simulink model "bms_final_sims_06"  (R2017b)
settings: Solver=VariableStepAuto  StartTime=0.0  StopTime=600  MaxStep=1e-4  RelTol=1e-3
undefined symbols (not defined in the file): DiscIntNeverNeededParam, Ion, Lithium, Ts_Control
libraries: powerlib x61, simulink x20, powerlib_meascontrol x3, simulink_extras x1, electricdrivelib x1
(part 2 of 2)

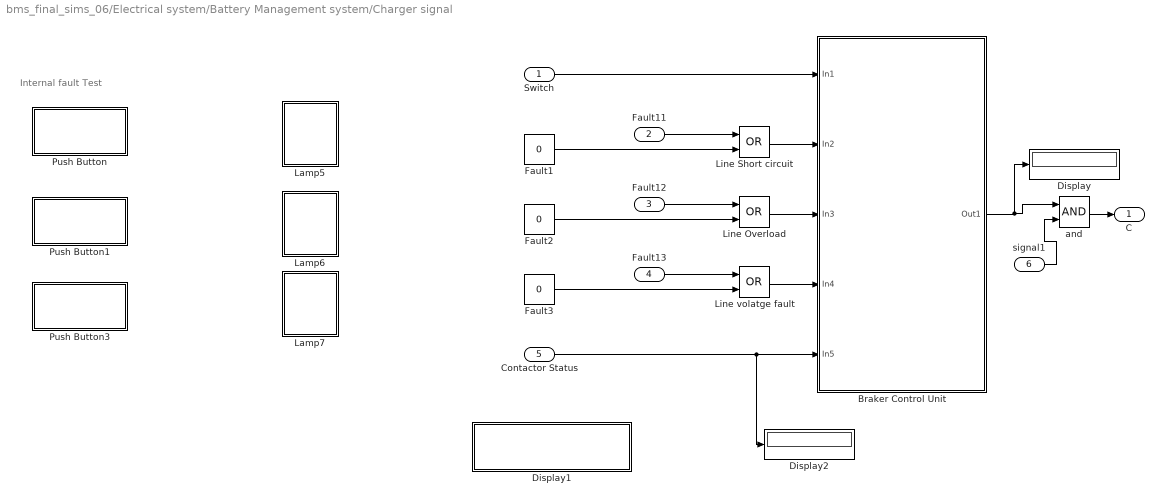
== system bms_final_sims_06/Electrical system/Battery Management system/Charger signal ==
  note: Internal fault Test
  Switch : Inport
  Fault11 : Inport  Port=2
  Fault12 : Inport  Port=3
  Fault13 : Inport  Port=4
  Contactor Status : Inport  Port=5
  signal1 : Inport  Port=6
  Braker Control Unit : Subsystem
  Display : Display
  Display1 : Subsystem  Description=Replaced Block  mask(Replaced Block){}
      mask help: This block has been replaced with an empty subsystem because it used functionality that is unavailable in Simulink R2016b.
      mask Display: fprintf('Replaced: %s\n','Dashboard Widget')
  Display2 : Display
  Fault1 : Constant  Value=0
  Fault2 : Constant  Value=0
  "Fault3 " : Constant  Value=0
  Lamp5 : Subsystem  DialogController=hmiCreateDDGDialog  IsWebBlock=on  mask(MWDashboardBlock){webBlockId=fb817cf7-7d11-4fa1-9a30-af3dbf48badf, webBlockType=lamp, ShowInLibBrowser=on, ShowInitialText=on, HMISrcModelName=bms_final_sims_06}
      mask prompts: webBlockType "WebBlock Type"; HMISrcModelName "Source Model"
      mask help: SimulinkHMI:dialogs:LampDialogDesc
      mask Help: helpview([docroot '/mapfiles/simulink.map'], 'hmi_lamp')
      mask Display:
      | if strcmp(get_param(bdroot(gcb),'BlockDiagramType'), 'library')
      |     image([(matlabroot) '/toolbox/simulink/hmi/icons/Lamp.png']);
      | end
  Lamp6 : Subsystem  DialogController=hmiCreateDDGDialog  IsWebBlock=on  mask(MWDashboardBlock){webBlockId=563e6533-b052-43b9-9c37-f49819595058, webBlockType=lamp, ShowInLibBrowser=on, ShowInitialText=on, HMISrcModelName=bms_final_sims_06}
      mask prompts: webBlockType "WebBlock Type"; HMISrcModelName "Source Model"
      mask help: SimulinkHMI:dialogs:LampDialogDesc
      mask Help: helpview([docroot '/mapfiles/simulink.map'], 'hmi_lamp')
      mask Display:
      | if strcmp(get_param(bdroot(gcb),'BlockDiagramType'), 'library')
      |     image([(matlabroot) '/toolbox/simulink/hmi/icons/Lamp.png']);
      | end
  Lamp7 : Subsystem  DialogController=hmiCreateDDGDialog  IsWebBlock=on  mask(MWDashboardBlock){webBlockId=1f8cf103-18fe-43eb-9390-d12ecce520ad, webBlockType=lamp, ShowInLibBrowser=on, ShowInitialText=on, HMISrcModelName=bms_final_sims_06}
      mask prompts: webBlockType "WebBlock Type"; HMISrcModelName "Source Model"
      mask help: SimulinkHMI:dialogs:LampDialogDesc
      mask Help: helpview([docroot '/mapfiles/simulink.map'], 'hmi_lamp')
      mask Display:
      | if strcmp(get_param(bdroot(gcb),'BlockDiagramType'), 'library')
      |     image([(matlabroot) '/toolbox/simulink/hmi/icons/Lamp.png']);
      | end
  Line Overload : Logic  Operator=OR  AllPortsSameDT=off  OutDataTypeStr=boolean
  Line Short circuit : Logic  Operator=OR  AllPortsSameDT=off  OutDataTypeStr=boolean
  Line volatge fault : Logic  Operator=OR  AllPortsSameDT=off  OutDataTypeStr=boolean
  Push Button : Subsystem  DialogController=hmiCreateDDGDialog  IsWebBlock=on  mask(MWDashboardBlock){webBlockId=7db8609d-5c17-4c61-9b24-8432e4b46d1c, webBlockType=pushbutton, ShowInLibBrwoser=on, ShowInitialText=on, HMISrcModelName=bms_final_sims_06}
      mask prompts: webBlockId "WebBlock Id"; webBlockType "WebBlock Type"; HMISrcModelName "Source Model"
      mask help: SimulinkHMI:dialogs:PushButtonDialogDesc
      mask Help: helpview([docroot '/mapfiles/simulink.map'], 'hmi_push_button')
      mask Display:
      | model = bdroot(gcb);
      | if strcmp(get_param(model,'BlockDiagramType'), 'library')
      |     image([(matlabroot) '/toolbox/simulink/hmi/icons/PushButton.png']);
      | end
  Push Button1 : Subsystem  DialogController=hmiCreateDDGDialog  IsWebBlock=on  mask(MWDashboardBlock){webBlockId=5bbde567-ebf7-4148-9d5e-f5393281e34a, webBlockType=pushbutton, ShowInLibBrwoser=on, ShowInitialText=on, HMISrcModelName=bms_final_sims_06}
      mask prompts: webBlockId "WebBlock Id"; webBlockType "WebBlock Type"; HMISrcModelName "Source Model"
      mask help: SimulinkHMI:dialogs:PushButtonDialogDesc
      mask Help: helpview([docroot '/mapfiles/simulink.map'], 'hmi_push_button')
      mask Display:
      | model = bdroot(gcb);
      | if strcmp(get_param(model,'BlockDiagramType'), 'library')
      |     image([(matlabroot) '/toolbox/simulink/hmi/icons/PushButton.png']);
      | end
  Push Button3 : Subsystem  DialogController=hmiCreateDDGDialog  IsWebBlock=on  mask(MWDashboardBlock){webBlockId=33bc8603-89d5-4b36-aa7c-12e4dfbd94cd, webBlockType=pushbutton, ShowInLibBrwoser=on, ShowInitialText=on, HMISrcModelName=bms_final_sims_06}
      mask prompts: webBlockId "WebBlock Id"; webBlockType "WebBlock Type"; HMISrcModelName "Source Model"
      mask help: SimulinkHMI:dialogs:PushButtonDialogDesc
      mask Help: helpview([docroot '/mapfiles/simulink.map'], 'hmi_push_button')
      mask Display:
      | model = bdroot(gcb);
      | if strcmp(get_param(model,'BlockDiagramType'), 'library')
      |     image([(matlabroot) '/toolbox/simulink/hmi/icons/PushButton.png']);
      | end
  and : Logic  AllPortsSameDT=off  OutDataTypeStr=boolean
  C : Outport
  wires:
  Switch/1 -> Braker Control Unit/1(In1)
  Braker Control Unit/1(Out1) -> and/1, Display/1
  Contactor Status/1 -> Display2/1, Braker Control Unit/5(In5)
  Line Short circuit/1 -> Braker Control Unit/2(In2)
  Line Overload/1 -> Braker Control Unit/3(In3)
  Line volatge fault/1 -> Braker Control Unit/4(In4)
  "Fault3 "/1 -> Line volatge fault/2
  Fault2/1 -> Line Overload/2
  Fault1/1 -> Line Short circuit/2
  Fault11/1 -> Line Short circuit/1
  Fault12/1 -> Line Overload/1
  Fault13/1 -> Line volatge fault/1
  and/1 -> C/1
  signal1/1 -> and/2

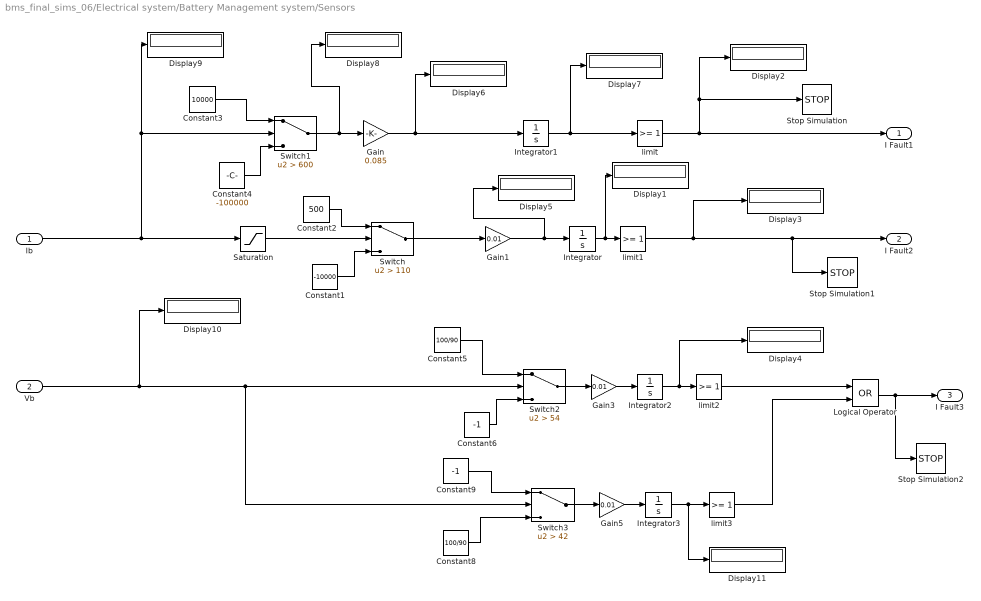
== system bms_final_sims_06/Electrical system/Battery Management system/Sensors ==
  Ib : Inport
  Vb : Inport  Port=2
  Constant1 : Constant  Value=-10000
  Constant2 : Constant  Value=500
  Constant3 : Constant  Value=10000
  Constant4 : Constant  Value=-100000
  Constant5 : Constant  Value=100/90
  Constant6 : Constant  Value=-1
  Constant8 : Constant  Value=100/90
  Constant9 : Constant  Value=-1
  Display{1..11} (11 alike) : Display
  Gain : Gain  Gain=0.085
  Gain1 : Gain  Gain=0.01
  Gain3 : Gain  Gain=0.01
  Gain5 : Gain  Gain=0.01
  Integrator{,1..3} (4 alike) : Integrator  LimitOutput=on  UpperSaturationLimit=1  LowerSaturationLimit=0
  Logical Operator : Logic  Operator=OR  AllPortsSameDT=off  OutDataTypeStr=boolean
  Saturation : Saturate  UpperLimit=600  LowerLimit=-1
  Stop Simulation : Stop
  Stop Simulation1 : Stop
  Stop Simulation2 : Stop
  Switch : Switch  Criteria=u2 > Threshold  Threshold=110
  Switch1 : Switch  Criteria=u2 > Threshold  Threshold=600
  Switch2 : Switch  Criteria=u2 > Threshold  Threshold=54
  Switch3 : Switch  Criteria=u2 > Threshold  Threshold=42
  limit{,1..3} (4 alike) : simulink/Logic and Bit Operations/Compare To Constant  relop=>=  const=1  OutDataTypeStr=boolean
  I Fault1 : Outport
  I Fault2 : Outport  Port=2
  I Fault3 : Outport  Port=3
  wires:
  limit/1 -> I Fault1/1, Stop Simulation/1, Display2/1
  limit1/1 -> Display3/1, I Fault2/1, Stop Simulation1/1
  Integrator/1 -> Display1/1, limit1/1
  Switch/1 -> Gain1/1
  Constant1/1 -> Switch/3
  Integrator1/1 -> Display7/1, limit/1
  Constant3/1 -> Switch1/1
  Gain1/1 -> Display5/1, Integrator/1
  Saturation/1 -> Switch/2
  Constant2/1 -> Switch/1
  Switch1/1 -> Display8/1, Gain/1
  Constant4/1 -> Switch1/3
  Ib/1 -> Saturation/1, Display9/1, Switch1/2
  Gain/1 -> Integrator1/1, Display6/1
  limit2/1 -> Logical Operator/1
  Constant8/1 -> Switch3/3
  Gain5/1 -> Integrator3/1
  Switch3/1 -> Gain5/1
  Integrator2/1 -> Display4/1, limit2/1
  Gain3/1 -> Integrator2/1
  Logical Operator/1 -> I Fault3/1, Stop Simulation2/1
  Switch2/1 -> Gain3/1
  Constant5/1 -> Switch2/1
  Constant6/1 -> Switch2/3
  Constant9/1 -> Switch3/1
  Vb/1 -> Display10/1, Switch3/2, Switch2/2
  Integrator3/1 -> Display11/1, limit3/1
  limit3/1 -> Logical Operator/2

== system bms_final_sims_06/Electrical system/Battery Pack/Battery Cell Equivalent ==
  t : Inport
  Battery : electricdrivelib/Extra Sources/Battery  BatType=Lithium-Ion  ShowTempParam=on  ThermalPreset=no  ShowAgeParam=off  NomV=48  NomQ=100  SOC=62.32  Batt_Tr=30  PresetModel=on  MaxQ=100  MinV=36  FullV=55.8714  Dis_rate=43.4783  R=0.0048  Normal_OP=90.4348  expZone="[51.8585      4.91304]"  current=[6.5 13 32.5]  Units=Time  Tci=20  NomT=20  T2=-30  MaxQ2=4.8  FullV2=7.1  Normal_OP2=5.655  expZone2="[6.58           1]"  Rca=0.6  ti=2000  Dp=0  Neq0=0  Tsim=1e6  Ta1=25  Qeol=5.4*0.9  Reol=0.013333*1.2  Char_age=[2.3478, 3]  Dis_age=[2.3478, 10]  N1=1500  N2=10500  N3=1000  N4=1400  Ta2=45  N5=950
  + : PMIOPort  Port=1  Side=Left
  - : PMIOPort  Port=2  Side=Left
  M : Outport
  wires:
  t/1 -> Battery/1
  Battery/1 -> M/1
  connections:
  Battery/LConn1 -- +/RConn1
  Battery/LConn2 -- -/RConn1

== system bms_final_sims_06/Electrical system/Dashboard Test/Total Fault Test ==
  note: External fault Test
  note: Internal fault Test
  Display : DisplayBlock  WebBlockId=825  ModelName=bms_final_sims_06  LabelPosition=Bottom  ShowInitialText=on  ShowFormattedStrings=off  Format=long  Alignment=Center
  Lamp : Subsystem  DialogController=hmiCreateDDGDialog  IsWebBlock=on  mask(MWDashboardBlock){webBlockId=fbdaa764-5bdc-4e5b-b7dd-49ea15c45a46, webBlockType=lamp, ShowInLibBrowser=on, ShowInitialText=on, HMISrcModelName=bms_final_sims_06}
      mask prompts: webBlockType "WebBlock Type"; HMISrcModelName "Source Model"
      mask help: SimulinkHMI:dialogs:LampDialogDesc
      mask Help: helpview([docroot '/mapfiles/simulink.map'], 'hmi_lamp')
      mask Display:
      | if strcmp(get_param(bdroot(gcb),'BlockDiagramType'), 'library')
      |     image([(matlabroot) '/toolbox/simulink/hmi/icons/Lamp.png']);
      | end
  Lamp1 : Subsystem  DialogController=hmiCreateDDGDialog  IsWebBlock=on  mask(MWDashboardBlock){webBlockId=082af06e-be4e-4919-b618-5f4e7f2fdde3, webBlockType=lamp, ShowInLibBrowser=on, ShowInitialText=on, HMISrcModelName=bms_final_sims_06}
      mask prompts: webBlockType "WebBlock Type"; HMISrcModelName "Source Model"
      mask help: SimulinkHMI:dialogs:LampDialogDesc
      mask Help: helpview([docroot '/mapfiles/simulink.map'], 'hmi_lamp')
      mask Display:
      | if strcmp(get_param(bdroot(gcb),'BlockDiagramType'), 'library')
      |     image([(matlabroot) '/toolbox/simulink/hmi/icons/Lamp.png']);
      | end
  Lamp2 : Subsystem  DialogController=hmiCreateDDGDialog  IsWebBlock=on  mask(MWDashboardBlock){webBlockId=516aa056-5fa7-4a7c-a023-c0dda198eca7, webBlockType=lamp, ShowInLibBrowser=on, ShowInitialText=on, HMISrcModelName=bms_final_sims_06}
      mask prompts: webBlockType "WebBlock Type"; HMISrcModelName "Source Model"
      mask help: SimulinkHMI:dialogs:LampDialogDesc
      mask Help: helpview([docroot '/mapfiles/simulink.map'], 'hmi_lamp')
      mask Display:
      | if strcmp(get_param(bdroot(gcb),'BlockDiagramType'), 'library')
      |     image([(matlabroot) '/toolbox/simulink/hmi/icons/Lamp.png']);
      | end
  Lamp3 : Subsystem  DialogController=hmiCreateDDGDialog  IsWebBlock=on  mask(MWDashboardBlock){webBlockId=fb978a94-c851-419f-aa5a-fdbf15f69119, webBlockType=lamp, ShowInLibBrowser=on, ShowInitialText=on, HMISrcModelName=bms_final_sims_06}
      mask prompts: webBlockType "WebBlock Type"; HMISrcModelName "Source Model"
      mask help: SimulinkHMI:dialogs:LampDialogDesc
      mask Help: helpview([docroot '/mapfiles/simulink.map'], 'hmi_lamp')
      mask Display:
      | if strcmp(get_param(bdroot(gcb),'BlockDiagramType'), 'library')
      |     image([(matlabroot) '/toolbox/simulink/hmi/icons/Lamp.png']);
      | end
  Lamp5 : Subsystem  DialogController=hmiCreateDDGDialog  IsWebBlock=on  mask(MWDashboardBlock){webBlockId=9848dc69-0a60-4163-96c5-d44da9eebd8e, webBlockType=lamp, ShowInLibBrowser=on, ShowInitialText=on, HMISrcModelName=bms_final_sims_06}
      mask prompts: webBlockType "WebBlock Type"; HMISrcModelName "Source Model"
      mask help: SimulinkHMI:dialogs:LampDialogDesc
      mask Help: helpview([docroot '/mapfiles/simulink.map'], 'hmi_lamp')
      mask Display:
      | if strcmp(get_param(bdroot(gcb),'BlockDiagramType'), 'library')
      |     image([(matlabroot) '/toolbox/simulink/hmi/icons/Lamp.png']);
      | end
  Lamp6 : Subsystem  DialogController=hmiCreateDDGDialog  IsWebBlock=on  mask(MWDashboardBlock){webBlockId=70f12f9c-07c1-4b6f-9ffa-b598c3129aa2, webBlockType=lamp, ShowInLibBrowser=on, ShowInitialText=on, HMISrcModelName=bms_final_sims_06}
      mask prompts: webBlockType "WebBlock Type"; HMISrcModelName "Source Model"
      mask help: SimulinkHMI:dialogs:LampDialogDesc
      mask Help: helpview([docroot '/mapfiles/simulink.map'], 'hmi_lamp')
      mask Display:
      | if strcmp(get_param(bdroot(gcb),'BlockDiagramType'), 'library')
      |     image([(matlabroot) '/toolbox/simulink/hmi/icons/Lamp.png']);
      | end
  Lamp7 : Subsystem  DialogController=hmiCreateDDGDialog  IsWebBlock=on  mask(MWDashboardBlock){webBlockId=49f89a92-cf53-4015-be2c-2362d2c7dbc5, webBlockType=lamp, ShowInLibBrowser=on, ShowInitialText=on, HMISrcModelName=bms_final_sims_06}
      mask prompts: webBlockType "WebBlock Type"; HMISrcModelName "Source Model"
      mask help: SimulinkHMI:dialogs:LampDialogDesc
      mask Help: helpview([docroot '/mapfiles/simulink.map'], 'hmi_lamp')
      mask Display:
      | if strcmp(get_param(bdroot(gcb),'BlockDiagramType'), 'library')
      |     image([(matlabroot) '/toolbox/simulink/hmi/icons/Lamp.png']);
      | end
  Push Button : Subsystem  DialogController=hmiCreateDDGDialog  IsWebBlock=on  mask(MWDashboardBlock){webBlockId=516cc25e-937b-498b-86c1-8ec3105bf36c, webBlockType=pushbutton, ShowInLibBrwoser=on, ShowInitialText=on, HMISrcModelName=bms_final_sims_06}
      mask prompts: webBlockId "WebBlock Id"; webBlockType "WebBlock Type"; HMISrcModelName "Source Model"
      mask help: SimulinkHMI:dialogs:PushButtonDialogDesc
      mask Help: helpview([docroot '/mapfiles/simulink.map'], 'hmi_push_button')
      mask Display:
      | model = bdroot(gcb);
      | if strcmp(get_param(model,'BlockDiagramType'), 'library')
      |     image([(matlabroot) '/toolbox/simulink/hmi/icons/PushButton.png']);
      | end
  Push Button1 : Subsystem  DialogController=hmiCreateDDGDialog  IsWebBlock=on  mask(MWDashboardBlock){webBlockId=e4ba1e2c-2ce9-46bd-ab8a-cd5544a9ea11, webBlockType=pushbutton, ShowInLibBrwoser=on, ShowInitialText=on, HMISrcModelName=bms_final_sims_06}
      mask prompts: webBlockId "WebBlock Id"; webBlockType "WebBlock Type"; HMISrcModelName "Source Model"
      mask help: SimulinkHMI:dialogs:PushButtonDialogDesc
      mask Help: helpview([docroot '/mapfiles/simulink.map'], 'hmi_push_button')
      mask Display:
      | model = bdroot(gcb);
      | if strcmp(get_param(model,'BlockDiagramType'), 'library')
      |     image([(matlabroot) '/toolbox/simulink/hmi/icons/PushButton.png']);
      | end
  Push Button2 : Subsystem  DialogController=hmiCreateDDGDialog  IsWebBlock=on  mask(MWDashboardBlock){webBlockId=76ac703d-c0e8-4889-a638-3fb074e42991, webBlockType=pushbutton, ShowInLibBrwoser=on, ShowInitialText=on, HMISrcModelName=bms_final_sims_06}
      mask prompts: webBlockId "WebBlock Id"; webBlockType "WebBlock Type"; HMISrcModelName "Source Model"
      mask help: SimulinkHMI:dialogs:PushButtonDialogDesc
      mask Help: helpview([docroot '/mapfiles/simulink.map'], 'hmi_push_button')
      mask Display:
      | model = bdroot(gcb);
      | if strcmp(get_param(model,'BlockDiagramType'), 'library')
      |     image([(matlabroot) '/toolbox/simulink/hmi/icons/PushButton.png']);
      | end
  Push Button3 : Subsystem  DialogController=hmiCreateDDGDialog  IsWebBlock=on  mask(MWDashboardBlock){webBlockId=c009c5cf-50ad-42da-a511-0218daf5ad02, webBlockType=pushbutton, ShowInLibBrwoser=on, ShowInitialText=on, HMISrcModelName=bms_final_sims_06}
      mask prompts: webBlockId "WebBlock Id"; webBlockType "WebBlock Type"; HMISrcModelName "Source Model"
      mask help: SimulinkHMI:dialogs:PushButtonDialogDesc
      mask Help: helpview([docroot '/mapfiles/simulink.map'], 'hmi_push_button')
      mask Display:
      | model = bdroot(gcb);
      | if strcmp(get_param(model,'BlockDiagramType'), 'library')
      |     image([(matlabroot) '/toolbox/simulink/hmi/icons/PushButton.png']);
      | end
  Push Button4 : Subsystem  DialogController=hmiCreateDDGDialog  IsWebBlock=on  mask(MWDashboardBlock){webBlockId=ca14451e-9a2a-4df3-9bee-2a5b308f3949, webBlockType=pushbutton, ShowInLibBrwoser=on, ShowInitialText=on, HMISrcModelName=bms_final_sims_06}
      mask prompts: webBlockId "WebBlock Id"; webBlockType "WebBlock Type"; HMISrcModelName "Source Model"
      mask help: SimulinkHMI:dialogs:PushButtonDialogDesc
      mask Help: helpview([docroot '/mapfiles/simulink.map'], 'hmi_push_button')
      mask Display:
      | model = bdroot(gcb);
      | if strcmp(get_param(model,'BlockDiagramType'), 'library')
      |     image([(matlabroot) '/toolbox/simulink/hmi/icons/PushButton.png']);
      | end
  Push Button5 : Subsystem  DialogController=hmiCreateDDGDialog  IsWebBlock=on  mask(MWDashboardBlock){webBlockId=16be5cf4-ca18-4a1e-93f1-989c159d4406, webBlockType=pushbutton, ShowInLibBrwoser=on, ShowInitialText=on, HMISrcModelName=bms_final_sims_06}
      mask prompts: webBlockId "WebBlock Id"; webBlockType "WebBlock Type"; HMISrcModelName "Source Model"
      mask help: SimulinkHMI:dialogs:PushButtonDialogDesc
      mask Help: helpview([docroot '/mapfiles/simulink.map'], 'hmi_push_button')
      mask Display:
      | model = bdroot(gcb);
      | if strcmp(get_param(model,'BlockDiagramType'), 'library')
      |     image([(matlabroot) '/toolbox/simulink/hmi/icons/PushButton.png']);
      | end
  Push Button6 : Subsystem  DialogController=hmiCreateDDGDialog  IsWebBlock=on  mask(MWDashboardBlock){webBlockId=fe97784f-3a2c-4507-b778-831998f088b7, webBlockType=pushbutton, ShowInLibBrwoser=on, ShowInitialText=on, HMISrcModelName=bms_final_sims_06}
      mask prompts: webBlockId "WebBlock Id"; webBlockType "WebBlock Type"; HMISrcModelName "Source Model"
      mask help: SimulinkHMI:dialogs:PushButtonDialogDesc
      mask Help: helpview([docroot '/mapfiles/simulink.map'], 'hmi_push_button')
      mask Display:
      | model = bdroot(gcb);
      | if strcmp(get_param(model,'BlockDiagramType'), 'library')
      |     image([(matlabroot) '/toolbox/simulink/hmi/icons/PushButton.png']);
      | end

== system bms_final_sims_06/Electrical system/Power Supply/Regulator  ==
  Vo : Inport
  Vref : Inport  Port=2
  PID : Subsystem
  Pulse Generator : Subsystem
  g1 : Outport
  g2 : Outport  Port=2
  wires:
  Vref/1 -> PID/2(Vref)
  Vo/1 -> PID/1(Vo)
  Pulse Generator/1(g1) -> g1/1
  Pulse Generator/2(g2) -> g2/1
  PID/1(Fs) -> Pulse Generator/1(Fs)

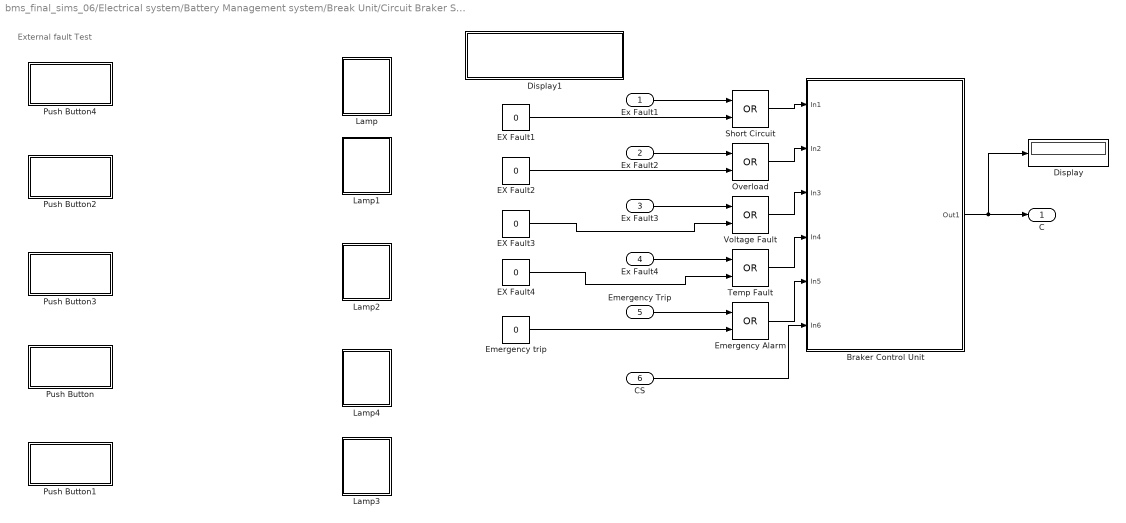
== system bms_final_sims_06/Electrical system/Battery Management system/Break Unit/Circuit Braker Signal ==
  note: External fault Test
  Ex Fault1 : Inport
  Ex Fault2 : Inport  Port=2
  Ex Fault3 : Inport  Port=3
  Ex Fault4 : Inport  Port=4
  Emergency Trip : Inport  Port=5
  CS : Inport  Port=6
  Braker Control Unit : Subsystem
  Display : Display
  Display1 : Subsystem  Description=Replaced Block  mask(Replaced Block){}
      mask help: This block has been replaced with an empty subsystem because it used functionality that is unavailable in Simulink R2016b.
      mask Display: fprintf('Replaced: %s\n','Dashboard Widget')
  "EX Fault1 " : Constant  Value=0
  "EX Fault2 " : Constant  Value=0
  EX Fault3 : Constant  Value=0
  EX Fault4 : Constant  Value=0
  Emergency Alarm : Logic  Operator=OR  AllPortsSameDT=off  OutDataTypeStr=boolean
  Emergency trip : Constant  Value=0
  Lamp : Subsystem  DialogController=hmiCreateDDGDialog  IsWebBlock=on  mask(MWDashboardBlock){webBlockId=301ec1c7-d5c1-44ad-a487-e42733662856, webBlockType=lamp, ShowInLibBrowser=on, ShowInitialText=on, HMISrcModelName=bms_final_sims_06}
      mask prompts: webBlockType "WebBlock Type"; HMISrcModelName "Source Model"
      mask help: SimulinkHMI:dialogs:LampDialogDesc
      mask Help: helpview([docroot '/mapfiles/simulink.map'], 'hmi_lamp')
      mask Display:
      | if strcmp(get_param(bdroot(gcb),'BlockDiagramType'), 'library')
      |     image([(matlabroot) '/toolbox/simulink/hmi/icons/Lamp.png']);
      | end
  Lamp1 : Subsystem  DialogController=hmiCreateDDGDialog  IsWebBlock=on  mask(MWDashboardBlock){webBlockId=9273cd8b-c478-425a-b7ce-52af7e70ffca, webBlockType=lamp, ShowInLibBrowser=on, ShowInitialText=on, HMISrcModelName=bms_final_sims_06}
      mask prompts: webBlockType "WebBlock Type"; HMISrcModelName "Source Model"
      mask help: SimulinkHMI:dialogs:LampDialogDesc
      mask Help: helpview([docroot '/mapfiles/simulink.map'], 'hmi_lamp')
      mask Display:
      | if strcmp(get_param(bdroot(gcb),'BlockDiagramType'), 'library')
      |     image([(matlabroot) '/toolbox/simulink/hmi/icons/Lamp.png']);
      | end
  Lamp2 : Subsystem  DialogController=hmiCreateDDGDialog  IsWebBlock=on  mask(MWDashboardBlock){webBlockId=6e0034b0-1bdf-4db9-bcc8-2229f749522d, webBlockType=lamp, ShowInLibBrowser=on, ShowInitialText=on, HMISrcModelName=bms_final_sims_06}
      mask prompts: webBlockType "WebBlock Type"; HMISrcModelName "Source Model"
      mask help: SimulinkHMI:dialogs:LampDialogDesc
      mask Help: helpview([docroot '/mapfiles/simulink.map'], 'hmi_lamp')
      mask Display:
      | if strcmp(get_param(bdroot(gcb),'BlockDiagramType'), 'library')
      |     image([(matlabroot) '/toolbox/simulink/hmi/icons/Lamp.png']);
      | end
  Lamp3 : Subsystem  DialogController=hmiCreateDDGDialog  IsWebBlock=on  mask(MWDashboardBlock){webBlockId=ee0838fd-836e-4035-9b30-b918c79ddf6f, webBlockType=lamp, ShowInLibBrowser=on, ShowInitialText=on, HMISrcModelName=bms_final_sims_06}
      mask prompts: webBlockType "WebBlock Type"; HMISrcModelName "Source Model"
      mask help: SimulinkHMI:dialogs:LampDialogDesc
      mask Help: helpview([docroot '/mapfiles/simulink.map'], 'hmi_lamp')
      mask Display:
      | if strcmp(get_param(bdroot(gcb),'BlockDiagramType'), 'library')
      |     image([(matlabroot) '/toolbox/simulink/hmi/icons/Lamp.png']);
      | end
  Lamp4 : Subsystem  DialogController=hmiCreateDDGDialog  IsWebBlock=on  mask(MWDashboardBlock){webBlockId=7b90d61e-1891-497c-8d5d-378f6a8e6971, webBlockType=lamp, ShowInLibBrowser=on, ShowInitialText=on, HMISrcModelName=bms_final_sims_06}
      mask prompts: webBlockType "WebBlock Type"; HMISrcModelName "Source Model"
      mask help: SimulinkHMI:dialogs:LampDialogDesc
      mask Help: helpview([docroot '/mapfiles/simulink.map'], 'hmi_lamp')
      mask Display:
      | if strcmp(get_param(bdroot(gcb),'BlockDiagramType'), 'library')
      |     image([(matlabroot) '/toolbox/simulink/hmi/icons/Lamp.png']);
      | end
  Overload : Logic  Operator=OR  AllPortsSameDT=off  OutDataTypeStr=boolean
  Push Button : Subsystem  DialogController=hmiCreateDDGDialog  IsWebBlock=on  mask(MWDashboardBlock){webBlockId=faa819ed-3f79-44e2-9171-4aa3daae911b, webBlockType=pushbutton, ShowInLibBrwoser=on, ShowInitialText=on, HMISrcModelName=bms_final_sims_06}
      mask prompts: webBlockId "WebBlock Id"; webBlockType "WebBlock Type"; HMISrcModelName "Source Model"
      mask help: SimulinkHMI:dialogs:PushButtonDialogDesc
      mask Help: helpview([docroot '/mapfiles/simulink.map'], 'hmi_push_button')
      mask Display:
      | model = bdroot(gcb);
      | if strcmp(get_param(model,'BlockDiagramType'), 'library')
      |     image([(matlabroot) '/toolbox/simulink/hmi/icons/PushButton.png']);
      | end
  Push Button1 : Subsystem  DialogController=hmiCreateDDGDialog  IsWebBlock=on  mask(MWDashboardBlock){webBlockId=c3a8ed2a-252d-4219-b454-98278993ce06, webBlockType=pushbutton, ShowInLibBrwoser=on, ShowInitialText=on, HMISrcModelName=bms_final_sims_06}
      mask prompts: webBlockId "WebBlock Id"; webBlockType "WebBlock Type"; HMISrcModelName "Source Model"
      mask help: SimulinkHMI:dialogs:PushButtonDialogDesc
      mask Help: helpview([docroot '/mapfiles/simulink.map'], 'hmi_push_button')
      mask Display:
      | model = bdroot(gcb);
      | if strcmp(get_param(model,'BlockDiagramType'), 'library')
      |     image([(matlabroot) '/toolbox/simulink/hmi/icons/PushButton.png']);
      | end
  Push Button2 : Subsystem  DialogController=hmiCreateDDGDialog  IsWebBlock=on  mask(MWDashboardBlock){webBlockId=3b173906-0574-4d26-a25f-9f7aaa039abe, webBlockType=pushbutton, ShowInLibBrwoser=on, ShowInitialText=on, HMISrcModelName=bms_final_sims_06}
      mask prompts: webBlockId "WebBlock Id"; webBlockType "WebBlock Type"; HMISrcModelName "Source Model"
      mask help: SimulinkHMI:dialogs:PushButtonDialogDesc
      mask Help: helpview([docroot '/mapfiles/simulink.map'], 'hmi_push_button')
      mask Display:
      | model = bdroot(gcb);
      | if strcmp(get_param(model,'BlockDiagramType'), 'library')
      |     image([(matlabroot) '/toolbox/simulink/hmi/icons/PushButton.png']);
      | end
  Push Button3 : Subsystem  DialogController=hmiCreateDDGDialog  IsWebBlock=on  mask(MWDashboardBlock){webBlockId=bed69022-b343-4a14-9e19-42c667cd160b, webBlockType=pushbutton, ShowInLibBrwoser=on, ShowInitialText=on, HMISrcModelName=bms_final_sims_06}
      mask prompts: webBlockId "WebBlock Id"; webBlockType "WebBlock Type"; HMISrcModelName "Source Model"
      mask help: SimulinkHMI:dialogs:PushButtonDialogDesc
      mask Help: helpview([docroot '/mapfiles/simulink.map'], 'hmi_push_button')
      mask Display:
      | model = bdroot(gcb);
      | if strcmp(get_param(model,'BlockDiagramType'), 'library')
      |     image([(matlabroot) '/toolbox/simulink/hmi/icons/PushButton.png']);
      | end
  Push Button4 : Subsystem  DialogController=hmiCreateDDGDialog  IsWebBlock=on  mask(MWDashboardBlock){webBlockId=086f9fe0-cb27-4f33-a126-3bf044f9497b, webBlockType=pushbutton, ShowInLibBrwoser=on, ShowInitialText=on, HMISrcModelName=bms_final_sims_06}
      mask prompts: webBlockId "WebBlock Id"; webBlockType "WebBlock Type"; HMISrcModelName "Source Model"
      mask help: SimulinkHMI:dialogs:PushButtonDialogDesc
      mask Help: helpview([docroot '/mapfiles/simulink.map'], 'hmi_push_button')
      mask Display:
      | model = bdroot(gcb);
      | if strcmp(get_param(model,'BlockDiagramType'), 'library')
      |     image([(matlabroot) '/toolbox/simulink/hmi/icons/PushButton.png']);
      | end
  Short Circuit : Logic  Operator=OR  AllPortsSameDT=off  OutDataTypeStr=boolean
  Temp Fault : Logic  Operator=OR  AllPortsSameDT=off  OutDataTypeStr=boolean
  Voltage Fault : Logic  Operator=OR  AllPortsSameDT=off  OutDataTypeStr=boolean
  C : Outport
  wires:
  Braker Control Unit/1(Out1) -> Display/1, C/1
  "EX Fault1 "/1 -> Short Circuit/2
  Ex Fault1/1 -> Short Circuit/1
  Short Circuit/1 -> Braker Control Unit/1(In1)
  Overload/1 -> Braker Control Unit/2(In2)
  Voltage Fault/1 -> Braker Control Unit/3(In3)
  Ex Fault2/1 -> Overload/1
  Emergency trip/1 -> Emergency Alarm/2
  Ex Fault3/1 -> Voltage Fault/1
  EX Fault3/1 -> Voltage Fault/2
  "EX Fault2 "/1 -> Overload/2
  Emergency Alarm/1 -> Braker Control Unit/5(In5)
  Temp Fault/1 -> Braker Control Unit/4(In4)
  Ex Fault4/1 -> Temp Fault/1
  Emergency Trip/1 -> Emergency Alarm/1
  EX Fault4/1 -> Temp Fault/2
  CS/1 -> Braker Control Unit/6(In6)

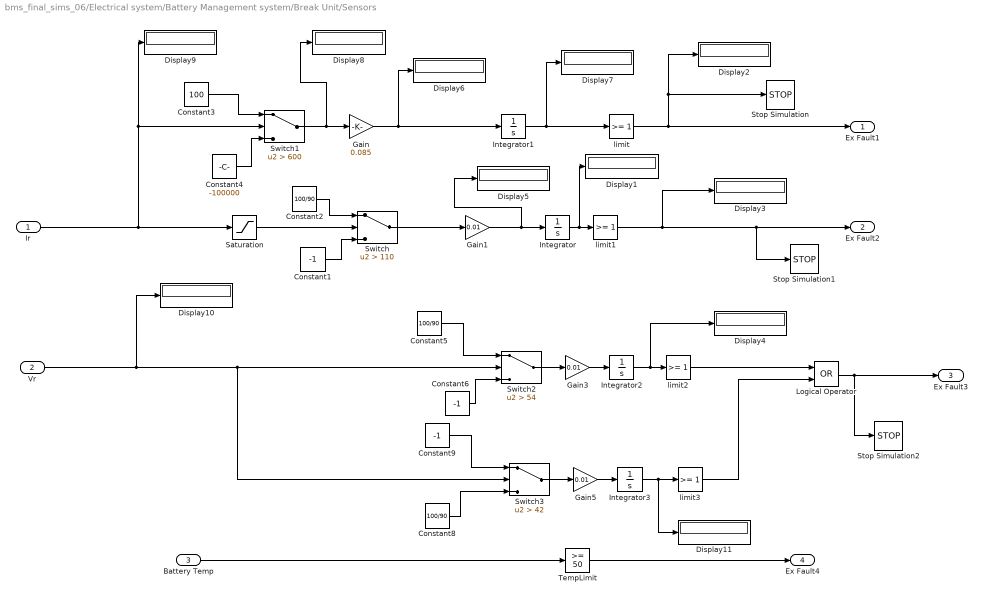
== system bms_final_sims_06/Electrical system/Battery Management system/Break Unit/Sensors ==
  Ir : Inport
  Vr : Inport  Port=2
  Battery Temp : Inport  Port=3
  Constant1 : Constant  Value=-1
  Constant2 : Constant  Value=100/90
  Constant3 : Constant  Value=100
  Constant4 : Constant  Value=-100000
  Constant5 : Constant  Value=100/90
  Constant6 : Constant  Value=-1
  Constant8 : Constant  Value=100/90
  Constant9 : Constant  Value=-1
  Display{1..11} (11 alike) : Display
  Gain : Gain  Gain=0.085
  Gain1 : Gain  Gain=0.01
  Gain3 : Gain  Gain=0.01
  Gain5 : Gain  Gain=0.01
  Integrator{,1..3} (4 alike) : Integrator  LimitOutput=on  UpperSaturationLimit=1  LowerSaturationLimit=0
  Logical Operator : Logic  Operator=OR  AllPortsSameDT=off  OutDataTypeStr=boolean
  Saturation : Saturate  UpperLimit=600  LowerLimit=-1
  Stop Simulation : Stop
  Stop Simulation1 : Stop
  Stop Simulation2 : Stop
  Switch : Switch  Criteria=u2 > Threshold  Threshold=110
  Switch1 : Switch  Criteria=u2 > Threshold  Threshold=600
  Switch2 : Switch  Criteria=u2 > Threshold  Threshold=54
  Switch3 : Switch  Criteria=u2 > Threshold  Threshold=42
  TempLimit : simulink/Logic and Bit Operations/Compare To Constant  relop=>=  const=50  OutDataTypeStr=boolean
  limit{,1..3} (4 alike) : simulink/Logic and Bit Operations/Compare To Constant  relop=>=  const=1  OutDataTypeStr=boolean
  Ex Fault1 : Outport
  Ex Fault2 : Outport  Port=2
  Ex Fault3 : Outport  Port=3
  Ex Fault4 : Outport  Port=4
  wires:
  limit1/1 -> Display3/1, Stop Simulation1/1, Ex Fault2/1
  Ir/1 -> Saturation/1, Display9/1, Switch1/2
  Gain/1 -> Integrator1/1, Display6/1
  Gain1/1 -> Display5/1, Integrator/1
  Integrator/1 -> Display1/1, limit1/1
  Switch/1 -> Gain1/1
  Switch1/1 -> Display8/1, Gain/1
  Constant4/1 -> Switch1/3
  Integrator1/1 -> Display7/1, limit/1
  Saturation/1 -> Switch/2
  Constant3/1 -> Switch1/1
  Constant2/1 -> Switch/1
  Constant1/1 -> Switch/3
  limit/1 -> Stop Simulation/1, Display2/1, Ex Fault1/1
  Battery Temp/1 -> TempLimit/1
  Logical Operator/1 -> Stop Simulation2/1, Ex Fault3/1
  Constant5/1 -> Switch2/1
  Constant6/1 -> Switch2/3
  Switch2/1 -> Gain3/1
  Gain3/1 -> Integrator2/1
  Integrator2/1 -> Display4/1, limit2/1
  Switch3/1 -> Gain5/1
  Gain5/1 -> Integrator3/1
  Vr/1 -> Display10/1, Switch3/2, Switch2/2
  Constant9/1 -> Switch3/1
  TempLimit/1 -> Ex Fault4/1
  Constant8/1 -> Switch3/3
  Integrator3/1 -> Display11/1, limit3/1
  limit2/1 -> Logical Operator/1
  limit3/1 -> Logical Operator/2

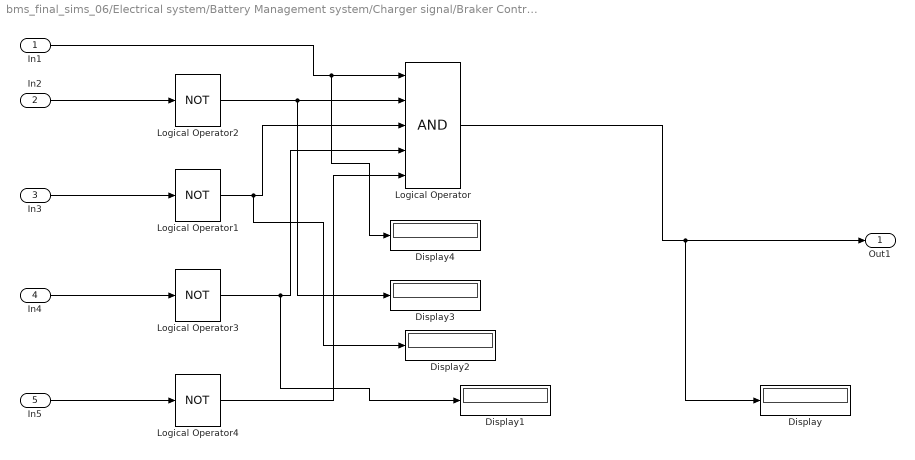
== system bms_final_sims_06/Electrical system/Battery Management system/Charger signal/Braker Control Unit ==
  In1 : Inport
  In2 : Inport  Port=2
  In3 : Inport  Port=3
  In4 : Inport  Port=4
  In5 : Inport  Port=5
  Display{,1..4} (5 alike) : Display
  Logical Operator : Logic  Inputs=5  AllPortsSameDT=off  OutDataTypeStr=boolean
  Logical Operator{1..4} (4 alike) : Logic  Operator=NOT  Inputs=4  AllPortsSameDT=off  OutDataTypeStr=boolean
  Out1 : Outport
  wires:
  Logical Operator4/1 -> Logical Operator/5
  Logical Operator3/1 -> Display1/1, Logical Operator/4
  Logical Operator1/1 -> Display2/1, Logical Operator/3
  Logical Operator2/1 -> Display3/1, Logical Operator/2
  In3/1 -> Logical Operator1/1
  In4/1 -> Logical Operator3/1
  In5/1 -> Logical Operator4/1
  Logical Operator/1 -> Out1/1, Display/1
  In1/1 -> Display4/1, Logical Operator/1
  In2/1 -> Logical Operator2/1

== system bms_final_sims_06/Electrical system/Battery Management system/Charger signal/Display1 ==

== system bms_final_sims_06/Electrical system/Battery Management system/Charger signal/Lamp5 ==

== system bms_final_sims_06/Electrical system/Battery Management system/Charger signal/Lamp6 ==

== system bms_final_sims_06/Electrical system/Battery Management system/Charger signal/Lamp7 ==

== system bms_final_sims_06/Electrical system/Battery Management system/Charger signal/Push Button ==

== system bms_final_sims_06/Electrical system/Battery Management system/Charger signal/Push Button1 ==

== system bms_final_sims_06/Electrical system/Battery Management system/Charger signal/Push Button3 ==

== system bms_final_sims_06/Electrical system/Dashboard Test/Total Fault Test/Lamp ==

== system bms_final_sims_06/Electrical system/Dashboard Test/Total Fault Test/Lamp1 ==

== system bms_final_sims_06/Electrical system/Dashboard Test/Total Fault Test/Lamp2 ==

== system bms_final_sims_06/Electrical system/Dashboard Test/Total Fault Test/Lamp3 ==

== system bms_final_sims_06/Electrical system/Dashboard Test/Total Fault Test/Lamp5 ==

== system bms_final_sims_06/Electrical system/Dashboard Test/Total Fault Test/Lamp6 ==

== system bms_final_sims_06/Electrical system/Dashboard Test/Total Fault Test/Lamp7 ==

== system bms_final_sims_06/Electrical system/Dashboard Test/Total Fault Test/Push Button ==

== system bms_final_sims_06/Electrical system/Dashboard Test/Total Fault Test/Push Button1 ==

== system bms_final_sims_06/Electrical system/Dashboard Test/Total Fault Test/Push Button2 ==

== system bms_final_sims_06/Electrical system/Dashboard Test/Total Fault Test/Push Button3 ==

== system bms_final_sims_06/Electrical system/Dashboard Test/Total Fault Test/Push Button4 ==

== system bms_final_sims_06/Electrical system/Dashboard Test/Total Fault Test/Push Button5 ==

== system bms_final_sims_06/Electrical system/Dashboard Test/Total Fault Test/Push Button6 ==

== system bms_final_sims_06/Electrical system/Power Supply/Regulator /PID ==
  Vo : Inport
  Vref : Inport  Port=2
  Discrete-Time Integrator : DiscreteIntegrator  InitialCondition=91.2e3  InitialConditionSetting=State (most efficient)  SampleTime=Ts_Control  LimitOutput=on  UpperSaturationLimit=300e3  LowerSaturationLimit=10e3  ICPrevOutput=DiscIntNeverNeededParam  ICPrevScaledInput=DiscIntNeverNeededParam
  Gain1 : Gain  Gain=500  SaturateOnIntegerOverflow=on  OutDataTypeStr=Inherit: Same as input  ParamDataTypeStr=Inherit: Same as input
  Gain4 : Gain  Gain=5e6  SaturateOnIntegerOverflow=on  OutDataTypeStr=Inherit: Same as input  ParamDataTypeStr=Inherit: Same as input
  Saturation1 : Saturate  UpperLimit=300e3  LowerLimit=10e3
  Sum1 : Sum  Inputs=|+-  SaturateOnIntegerOverflow=on  InputSameDT=on  OutDataTypeStr=Inherit: Same as first input
  Sum2 : Sum  SaturateOnIntegerOverflow=on  InputSameDT=on  OutDataTypeStr=Inherit: Same as first input
  Fs : Outport
  wires:
  Vo/1 -> Sum1/1
  Vref/1 -> Sum1/2
  Sum1/1 -> Gain1/1, Gain4/1
  Gain4/1 -> Discrete-Time Integrator/1
  Discrete-Time Integrator/1 -> Sum2/2
  Sum2/1 -> Saturation1/1
  Gain1/1 -> Sum2/1
  Saturation1/1 -> Fs/1

== system bms_final_sims_06/Electrical system/Power Supply/Regulator /Pulse Generator ==
  Fs : Inport
  Constant1 : Constant  Value=0.5
  Data Type Conversion1 : DataTypeConversion  OutDataTypeStr=double
  Fcn : Fcn  Expr=0.5 * ( u(1)+1 )
  Gain1 : Gain  Gain=2/pi  SaturateOnIntegerOverflow=on  OutDataTypeStr=Inherit: Same as input  ParamDataTypeStr=Inherit: Same as input
  Gain2 : Gain  Gain=2*pi  SaturateOnIntegerOverflow=on  OutDataTypeStr=Inherit: Same as input  ParamDataTypeStr=Inherit: Same as input
  Integrator : Integrator
  Logical Operator : Logic  Operator=NOT  AllPortsSameDT=off  OutDataTypeStr=float('double')
  Relational Operator : RelationalOperator  OutDataTypeStr=boolean  RndMeth=Nearest
  Trigonometric Function : Trigonometry  Operator=asin
  Trigonometric Function3 : Trigonometry
  g1 : Outport
  g2 : Outport  Port=2
  tag scope: Fs=global
  wires:
  Fs/1 -> Gain2/1, [Fs]
  Gain2/1 -> Integrator/1
  Data Type Conversion1/1 -> g1/1
  Logical Operator/1 -> g2/1
  Fcn/1 -> Relational Operator/2
  Relational Operator/1 -> Logical Operator/1, Data Type Conversion1/1
  Constant1/1 -> Relational Operator/1
  Integrator/1 -> Trigonometric Function3/1
  Trigonometric Function/1 -> Gain1/1
  Gain1/1 -> Fcn/1
  Trigonometric Function3/1 -> Trigonometric Function/1

== system bms_final_sims_06/Electrical system/Battery Management system/Break Unit/Circuit Braker Signal/Braker Control Unit ==
  In1 : Inport
  In2 : Inport  Port=2
  In3 : Inport  Port=3
  In4 : Inport  Port=4
  In5 : Inport  Port=5
  In6 : Inport  Port=6
  Logical Operator : Logic  Inputs=6  AllPortsSameDT=off  OutDataTypeStr=boolean
  Logical Operator{1..5} (5 alike) : Logic  Operator=NOT  Inputs=4  AllPortsSameDT=off  OutDataTypeStr=boolean
  Out1 : Outport
  wires:
  Logical Operator1/1 -> Logical Operator/3
  Logical Operator2/1 -> Logical Operator/2
  In3/1 -> Logical Operator1/1
  Logical Operator/1 -> Out1/1
  In2/1 -> Logical Operator2/1
  In1/1 -> Logical Operator4/1
  Logical Operator4/1 -> Logical Operator/1
  Logical Operator3/1 -> Logical Operator/5
  Logical Operator5/1 -> Logical Operator/4
  In4/1 -> Logical Operator5/1
  In5/1 -> Logical Operator3/1
  In6/1 -> Logical Operator/6

== system bms_final_sims_06/Electrical system/Battery Management system/Break Unit/Circuit Braker Signal/Display1 ==

== system bms_final_sims_06/Electrical system/Battery Management system/Break Unit/Circuit Braker Signal/Lamp ==

== system bms_final_sims_06/Electrical system/Battery Management system/Break Unit/Circuit Braker Signal/Lamp1 ==

== system bms_final_sims_06/Electrical system/Battery Management system/Break Unit/Circuit Braker Signal/Lamp2 ==

== system bms_final_sims_06/Electrical system/Battery Management system/Break Unit/Circuit Braker Signal/Lamp3 ==

== system bms_final_sims_06/Electrical system/Battery Management system/Break Unit/Circuit Braker Signal/Lamp4 ==

== system bms_final_sims_06/Electrical system/Battery Management system/Break Unit/Circuit Braker Signal/Push Button ==

== system bms_final_sims_06/Electrical system/Battery Management system/Break Unit/Circuit Braker Signal/Push Button1 ==

== system bms_final_sims_06/Electrical system/Battery Management system/Break Unit/Circuit Braker Signal/Push Button2 ==

== system bms_final_sims_06/Electrical system/Battery Management system/Break Unit/Circuit Braker Signal/Push Button3 ==

== system bms_final_sims_06/Electrical system/Battery Management system/Break Unit/Circuit Braker Signal/Push Button4 ==

== matlab function bms_final_sims_06/Electrical system/Battery Management system/ function/MATLAB Function1 ==
  data: I input; Iavg output; w input; wavg output
function [Iavg,wavg] = avg_fcn(I,w)
Iavg=0;
wavg=0;
while(1) 
    for i=1:180
        Iav=((Iavg*(i-1))+I)/i;
        wav=((wavg*(i-1))+w)/i;
        pause(1);
    end
    i=1;
    Iavg=Iav;
    wavg=wav;
end   
y = u;

== matlab function bms_final_sims_06/Electrical system/Battery Management system/ function/MATLAB Function ==
  data: soc input; soh output
function soh = soc_fcn(soc)
n=3500;
ds=diff(soc);
time=0:1e-03:600;
dt=diff(time);
c=0,u=0,d=0;
if ds/dt>0 && soc>80
    u=1;
    if d=1
        c=c+1;
        u=0;
    end
    d=0;
end
elif ds/dt<0 && soc<20
    d=1;
    if u=1
        c=c+1;
        d=0;
    end
    u=0;
end
soh=(c/n)*100;
y = u;

== matlab function bms_final_sims_06/Electrical system/Battery Management system/ function/MATLAB Function2 ==
  data: Iavg input; R output; S input; wavg input
function R = range_fcn(Iavg,S,wavg)
while (1)
    t=S/Iavg;
    rad=0.35;
    V=rad*wavg;
    R=t*V;
    pause(180);
end
y = u;
